simulink model "Pur_Pursuit"  (R2022a)
settings: Solver=FixedStepAuto  StartTime=0.0  StopTime=T  FixedStep=Te  RelTol=1e-3
undefined symbols (not defined in the file or in its folder): d, DiscIntNeverNeededParam, L, psi, v
libraries: vehdynlibsteering x2, robotmobilelib x1, simulink x1
settings Model: Creator=leonj  LastModifiedBy=leonj

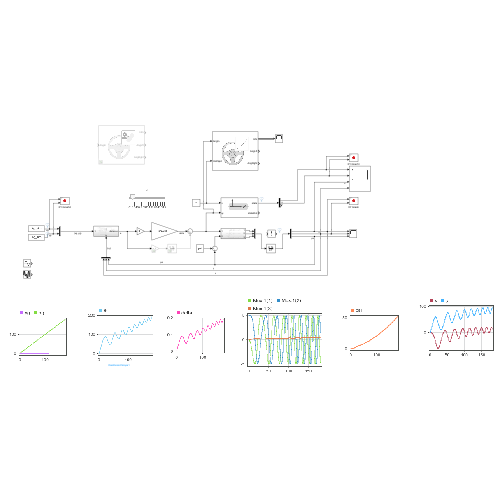
[thumbnail: Simulink's stored preview of the top-level diagram]
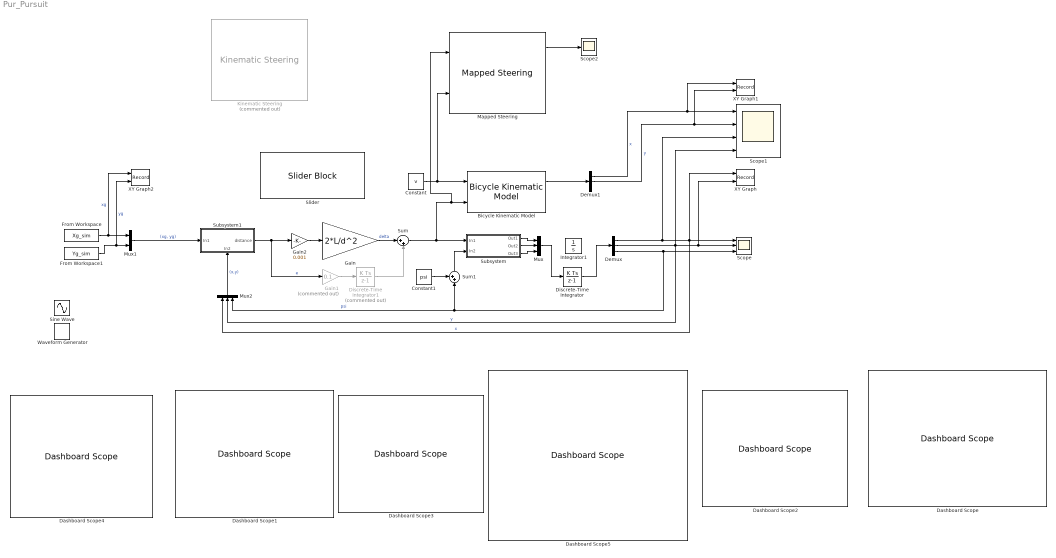
== system Pur_Pursuit ==
  Bicycle Kinematic Model : robotmobilelib/Bicycle Kinematic Model  VehicleInputs=Vehicle Speed & Steering Angle  WheelBase=1  VehicleSpeedRange=[-inf inf]  MaxSteeringAngle=pi/4  InitialState=[0; 0; 0]  SimulateUsing=Interpreted execution
      settings: SourceProductBaseCode=RO
  Constant : Constant  Value=v
  Constant1 : Constant  Value=psi
  Dashboard Scope : DashboardScope  Ymin=0  Ymax=10
  Dashboard Scope1 : DashboardScope  Ymin=0  Ymax=20
  Dashboard Scope2 : DashboardScope  Ymax=40
  Dashboard Scope3 : DashboardScope
  Dashboard Scope4 : DashboardScope  Ymin=-10  Ymax=10
  Dashboard Scope5 : DashboardScope
  Demux : Demux  Outputs=3
  Demux1 : Demux  Outputs=3
  Discrete-Time Integrator : DiscreteIntegrator  SampleTime=-1  ICPrevOutput=DiscIntNeverNeededParam  ICPrevScaledInput=DiscIntNeverNeededParam
  Discrete-Time Integrator1 : DiscreteIntegrator  Commented=on  SampleTime=-1  ICPrevOutput=DiscIntNeverNeededParam  ICPrevScaledInput=DiscIntNeverNeededParam
  From Workspace : FromWorkspace  VariableName=Xg_sim
  From Workspace1 : FromWorkspace  VariableName=Yg_sim
  Gain : Gain  Gain=2*L/d^2
  Gain1 : Gain  Commented=on  Gain=0.1
  Gain2 : Gain  Gain=0.001
  Integrator1 : Integrator
  Kinematic Steering : vehdynlibsteering/Kinematic Steering  Commented=on  StrgType=Rack and pinion  StrgRatioType=Constant  Loc=Front  NrmlFctr=0.01  TrckWdth=1  WhlBase=1.524  Db=0  StrgRng=1.25*pi  StrgAngBpts="[-6.2832   -5.0265   -3.7699   -2.5133   -1.2566         0    1.2566    2.5133    3.7699    5.0265    6.2832]"  StrgRatioTbl=|  StrgRatio=100  PctAckIn=off  PctAck=100  PctAckTbl=ones(1,11)*100  StrgArmLngth=0.1  RckCsLngth=0.5  TieRodLngth=0.248  D=0.2  PnnRadius=0.00085818  PnnRadiusTbl="[0.0055    0.0055    0.0056    0.0057    0.0058    0.0057    0.0057    0.0057    0.0056    0.0055    0.0055]"  RodLngth=0.1  ParaArmLngth=0.9  aMode=2
      | [13.5000   13.3750   13.2500   13.1250   13.0000   13.0000   13.0000   13.1250   13.2500   13.3750   13.5000
      | ]
  Mapped Steering : vehdynlibsteering/Mapped Steering  SpdDpd=on  IndexType=Steering wheel angle  GrType=Constant  StrgAngBpts=[-1.5*pi -0.72*pi -0.17*pi 0.17*pi 0.72*pi 1.5*pi]  RackDispBpts=[-40 -19.2 -4.53 4.53 19.2 40]  Gr=8.28*2*pi  GrTbl=[9.87 9.87 7.16 7.16 9.87 9.87]*2*pi  WhlLftTbl=[-1.5*pi -0.72*pi -0.17*pi 0.17*pi 0.72*pi 1.5*pi]/13.5  WhlRghtTbl=[-1.5*pi -0.72*pi -0.17*pi 0.17*pi 0.72*pi 1.5*pi]/13.5  VehSpdBpts=[-1 1]  SpdFctTbl=[1 1]  aMode=2
      settings: SourceProductBaseCode=VE
  Mux : Mux  Inputs=3
  Mux1 : Mux  Inputs=2
  Mux2 : Mux  Inputs=3
  Scope : Scope  NumInputPorts=3
  Scope1 : Scope  NumInputPorts=4
  Scope2 : Scope
  Sine Wave : Sin  SampleTime=0
  Slider : SliderBlock  ScaleMax=20  TickInterval=1
  Subsystem : Subsystem
  Subsystem1 : Subsystem
      settings: PortSchema="{\"entries\":[{\"content\":{\"sides\":[{\"content\":{\"connectorIds\":[\"In1\"]},\"type\":\"ConnectorPlacement.EquallySpacedRectSide\",\"uuid\":\"ce90e960-11cd-4418-99a1-1b66fd5dbedd\"},{\"content\":{\"connectorIds\":[\"Out1\"],\"side\":\"RIGHT\"},\"type\":\"ConnectorPlacement.EquallySpacedRectSide\",\"uuid\":\"4009b7ba-f23e-4f4f-83b3-155686f470f1\"},{\"content\":{\"connectorIds\":[],\"side\":\"TOP\"},\"type\":\"ConnectorPlacement.EquallySpacedRectSide\",\"uuid\":\"b80a7d2e-b613-4108-bb82-78c415c4d804\"},{\"content\":{\"connectorIds\":[\"In2\"],\"side\":\"BOTTOM\"},\"type\":\"ConnectorPlacement.EquallySpacedRectSide\",\"uuid\":\"a8b029d2-5aaf-4a5a-b207-d511f0229fe7\"}]},\"type\":\"ConnectorPlacement.EquallySpacedConnector\",\"uuid\":\"491b8389-c1b4-4f5d-bd99-aaa20e708be7\"}],\"packageUris\":[\"http://schema.mathworks.com/mf0/Connector/R2020b\"],\"version\":\"1.0\"}"
  Sum : Sum  Inputs=|++
  Sum1 : Sum  Inputs=++|
  Waveform Generator : simulink/Sources/Waveform Generator  OutMin=[]  OutMax=[]  OutDataTypeStr=double  SelectedSignal=1  BlockNames=MultiportSwitch_e3df3653d217406  SampleTime=0.1
  XY Graph : Record  FileSettingsInternal="{\"entries\":[{\"content\":{\"excelSettings\":{\"content\":{},\"type\":\"Streamout.ExcelSettings\"}},\"type\":\"Streamout.FileSettingStorage\",\"uuid\":\"9e7d6c22-062b-43a1-8a36-f0f4a7b8e0a7\"}],\"packageUris\":[\"http://schema.mathworks.com/mf0/streamout_blocks/R2020a\"],\"version\":\"1.0\"}"  Layout=[1 1]  SignalsInternal="{\"entries\":[{\"content\":{\"signals\":[{\"content\":{\"blockPath\":[\"Pur_Pursuit/XY Graph\"],\"channel\":[],\"dimensions\":[1],\"domain\":\"Pur_Pursuit/XY Graph\",\"lineColor\":\"#ff13a6\",\"plots\":[],\"port\":1,\"sid\":[\"\"],\"signalID\":56877,\"signalName\":\"x\"},\"type\":\"RecordBlkView.Signal\",\"uuid\":\"fae13afb-41f6-4e89-a0bc-626496c26790\"},{\"content\":{\"blockPath\":[\"Pur_Pursuit/XY Graph\"],\"channel\":[],\"dimensions\":[1],\"domain\":\"Pur_Pursuit/XY Graph\",\"lineColor\":\"#fe330a\",\"plots\":[],\"port\":2,\"sid\":[\"\"],\"signalID\":56881,\"signalName\":\"y\"},\"type\":\"RecordBlkView.Signal\",\"uuid\":\"fb334447-fae1-4bff-8087-0e1c41a3958b\"}]},\"type\":\"RecordBlkView.InputSignals\",\"uuid\":\"6adf6ab7-89cd-4d09-a430-2e8164cf3a85\"}],\"packageUris\":[\"http://schema.mathworks.com/mf0/streamout_blocks/R2020a\"],\"version\":\"1.0\"}"  VisualizationBindings="{\"xyplotplugin\":{\"info\":[{\"series\":[],\"subplotID\":1},{\"series\":[],\"subplotID\":9}]}}"  CompatibilityTag=XY
  XY Graph1 : Record  FileSettingsInternal="{\"entries\":[{\"content\":{\"excelSettings\":{\"content\":{},\"type\":\"Streamout.ExcelSettings\"}},\"type\":\"Streamout.FileSettingStorage\",\"uuid\":\"47e1d91c-023c-4af7-99e1-4cf7285ac6c4\"}],\"packageUris\":[\"http://schema.mathworks.com/mf0/streamout_blocks/R2020a\"],\"version\":\"1.0\"}"  Layout=[1 1]  SignalsInternal="{\"entries\":[{\"content\":{\"signals\":[{\"content\":{\"blockPath\":[\"Pur_Pursuit/XY Graph1\"],\"channel\":[],\"dimensions\":[1],\"domain\":\"Pur_Pursuit/XY Graph1\",\"lineColor\":\"#22b573\",\"plots\":[],\"port\":1,\"sid\":[\"\"],\"signalID\":56885,\"signalName\":\"x\"},\"type\":\"RecordBlkView.Signal\",\"uuid\":\"03cb08e9-1d5d-4078-954b-7a6d3c831847\"},{\"content\":{\"blockPath\":[\"Pur_Pursuit/XY Graph1\"],\"channel\":[],\"dimensions\":[1],\"domain\":\"Pur_Pursuit/XY Graph1\",\"lineColor\":\"#0072bd\",\"plots\":[],\"port\":2,\"sid\":[\"\"],\"signalID\":56889,\"signalName\":\"y\"},\"type\":\"RecordBlkView.Signal\",\"uuid\":\"5de7a3e2-01d6-46d1-aba3-03d38796b132\"}]},\"type\":\"RecordBlkView.InputSignals\",\"uuid\":\"464cd8ba-4689-43bd-b3d3-96e7317aec6e\"}],\"packageUris\":[\"http://schema.mathworks.com/mf0/streamout_blocks/R2020a\"],\"version\":\"1.0\"}"  VisualizationBindings="{\"xyplotplugin\":{\"info\":[{\"series\":[],\"subplotID\":1}]}}"  CompatibilityTag=XY
  XY Graph2 : Record  FileSettingsInternal="{\"entries\":[{\"content\":{\"excelSettings\":{\"content\":{},\"type\":\"Streamout.ExcelSettings\"}},\"type\":\"Streamout.FileSettingStorage\",\"uuid\":\"e09d139c-0e52-4774-8a8f-f40d80492498\"}],\"packageUris\":[\"http://schema.mathworks.com/mf0/streamout_blocks/R2020a\"],\"version\":\"1.0\"}"  Layout=[1 1]  SignalsInternal="{\"entries\":[{\"content\":{\"signals\":[{\"content\":{\"blockPath\":[\"Pur_Pursuit/XY Graph2\"],\"channel\":[],\"dimensions\":[1],\"domain\":\"Pur_Pursuit/XY Graph2\",\"lineColor\":\"#d95319\",\"plots\":[],\"port\":1,\"sid\":[\"\"],\"signalID\":56893,\"signalName\":\"xg\"},\"type\":\"RecordBlkView.Signal\",\"uuid\":\"91a9ea4d-1692-44ef-8585-96635eb44551\"},{\"content\":{\"blockPath\":[\"Pur_Pursuit/XY Graph2\"],\"channel\":[],\"dimensions\":[1],\"domain\":\"Pur_Pursuit/XY Graph2\",\"lineColor\":\"#edb120\",\"plots\":[],\"port\":2,\"sid\":[\"\"],\"signalID\":56897,\"signalName\":\"yg\"},\"type\":\"RecordBlkView.Signal\",\"uuid\":\"704dd878-ffe5-40a3-9e46-9e748ec4903e\"}]},\"type\":\"RecordBlkView.InputSignals\",\"uuid\":\"e7cbe83e-159b-48a2-85ec-73bed0dddff1\"}],\"packageUris\":[\"http://schema.mathworks.com/mf0/streamout_blocks/R2020a\"],\"version\":\"1.0\"}"  VisualizationBindings="{\"xyplotplugin\":{\"info\":[{\"series\":[],\"subplotID\":1}]}}"  CompatibilityTag=XY
  wires:
  Mux2/1 -> Subsystem1/2(In2)  "(x,y)"
  Demux/1 -> Mux2/1, XY Graph/1, Scope/1, Scope1/3  "x"
  From Workspace/1 -> XY Graph2/1, Mux1/1  "xg"
  Subsystem/2(Out2) -> Mux/2
  Demux/2 -> Mux2/2, Scope1/4, XY Graph/2, Scope/2  "y"
  Mux1/1 -> Subsystem1/1(In1)  "(xg, yg)"
  From Workspace1/1 -> XY Graph2/2, Mux1/2  "yg"
  Subsystem/1(Out1) -> Mux/1
  Demux/3 -> Sum1/2, Mux2/3, Scope/3  "psi"
  Subsystem/3(Out3) -> Mux/3
  Subsystem1/1(distance) -> Gain2/1, Gain1/1  "e"
  Gain1/1 -> Discrete-Time Integrator1/1
  Gain/1 -> Sum/1  "delta"
  Sum/1 -> Mapped Steering/1, Bicycle Kinematic Model/2, Subsystem/1(In1)
  Constant/1 -> Bicycle Kinematic Model/1, Mapped Steering/2
  Bicycle Kinematic Model/1 -> Demux1/1
  Demux1/1 -> XY Graph1/1, Scope1/1  "x"
  Demux1/2 -> XY Graph1/2, Scope1/2  "y"
  Mux/1 -> Discrete-Time Integrator/1
  Discrete-Time Integrator/1 -> Demux/1
  Discrete-Time Integrator1/1 -> Sum/2
  Gain2/1 -> Gain/1
  Mapped Steering/1 -> Scope2/1
  Sum1/1 -> Subsystem/2(In2)
  Constant1/1 -> Sum1/1

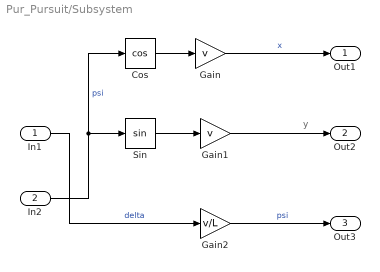
== system Pur_Pursuit/Subsystem ==
  note: y
  In1 : Inport
  In2 : Inport  Port=2
  Cos : Trigonometry  Operator=cos
  Gain : Gain  Gain=v
  Gain1 : Gain  Gain=v
  Gain2 : Gain  Gain=v/L
  Sin : Trigonometry
  Out1 : Outport
  Out2 : Outport  Port=2
  Out3 : Outport  Port=3
  wires:
  Cos/1 -> Gain/1
  Gain/1 -> Out1/1  "x"
  Sin/1 -> Gain1/1
  Gain1/1 -> Out2/1
  In2/1 -> Sin/1, Cos/1  "psi"
  In1/1 -> Gain2/1  "delta"
  Gain2/1 -> Out3/1  "psi"

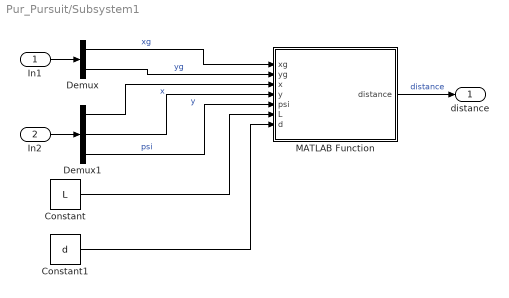
== system Pur_Pursuit/Subsystem1 ==
  In1 : Inport
  In2 : Inport  Port=2
  Constant : Constant  Value=L
  Constant1 : Constant  Value=d
  Demux : Demux  Outputs=2
  Demux1 : Demux  Outputs=3
  MATLAB Function : MATLAB Function  TreatAsAtomicUnit=on
  distance : Outport
  wires:
  MATLAB Function/1(distance) -> distance/1  "distance"
  In1/1 -> Demux/1
  In2/1 -> Demux1/1
  Demux1/2 -> MATLAB Function/4(y)  "y"
  Demux/2 -> MATLAB Function/2(yg)  "yg"
  Demux1/1 -> MATLAB Function/3(x)  "x"
  Demux/1 -> MATLAB Function/1(xg)  "xg"
  Demux1/3 -> MATLAB Function/5(psi)  "psi"
  Constant/1 -> MATLAB Function/6(L)
  Constant1/1 -> MATLAB Function/7(d)

== matlab function Pur_Pursuit/Subsystem1/MATLAB Function ==
  data: xg input; distance output; yg input; x input; y input; psi input; L input; d input
function distance  = differentiel(xg,yg,x,y,psi,L,d)
%UNTITLED2 Summary of this function goes here
%   Detailed explanation goes here
% distance = sqrt( ...
%     (xg-(x-0.5*L+d)*cos(psi))^2 ...
%     +(yg-(y-0.5*L+d)*sin(psi))^2 ...
%     );

distance = norm([xg yg]-[x+(0.5*L-d)*sin(psi) y+(-0.5*L+d)*cos(psi)]);
end
